simulink model "Lab2_3_sol"  (R2023b)
settings: Solver=VariableStepDiscrete  StartTime=0.0  StopTime=256*256*2  RelTol=1e-3  EnableMultiTasking=on
PreLoadFcn:
  | ImSize = 256;
undefined symbols (not defined in the file): gray, xc7k325tfbg676
libraries: hdlBasic x31, dspsigattribs x5, visionsources x1, vmcUtilities x1
settings Model: Creator=arvinds  LastModifiedBy=robg
settings SolverCC: AlgebraicLoopSolver=TrustRegion
settings DataIOCC: LimitDataPoints=on  SaveFormat=Array  SignalLoggingSaveFormat=ModelDataLogs  ReturnWorkspaceOutputs=off
settings OptimizationCC: ExpressionDepthLimit=2147483647  LifeSpan=inf
settings DebuggingCC: UnderspecifiedInitializationDetection=Classic  MergeDetectMultiDrivingBlocksExec=none  SolverPrmCheckMsg=warning  FcnCallInpInsideContextMsg=warning  UnconnectedInputMsg=warning  UnconnectedOutputMsg=warning  UnconnectedLineMsg=warning  AllowSymbolicDim=off  StateNameClashWarn=warning  SFUnexpectedBacktrackingDiag=warning  SFNoUnconditionalDefaultTransitionDiag=warning  SFExecutionAtInitializationDiag=none  ArithmeticOperatorsInVariantConditions=warning
settings HardwareCC: ProdBitPerPointer=32  ProdBitPerSizeT=32  ProdBitPerPtrDiffT=32  ProdLargestAtomicFloat=None  ProdIntDivRoundTo=Undefined  ProdEndianess=Unspecified  ProdWordSize=32  ProdHWDeviceType=32-bit Generic
settings ModelReferenceCC: EnableRefExpFcnMdlSchedulingChecks=on  PropagateSignalLabelsOutOfModel=off
settings SFSimCC: SimUseLocalCustomCode=off  CustomCodeUndefinedFunction=UseInterfaceOnly
settings RTWCC: RTWUseLocalCustomCode=off  DLArmComputeVersion=19.05
settings CodeAppCC: StateflowObjectComments=on
settings GRTTargetCC: TargetLangStandard=C89/C90 (ANSI)  CombineOutputUpdateFcns=off  GRTInterface=on
settings ConfigComp: CovMetricSettings=dw  CovSaveCumulativeToWorkspaceVar=on  CovSaveSingleToWorkspaceVar=on  CovExternalEMLEnable=off  CovSFcnEnable=off

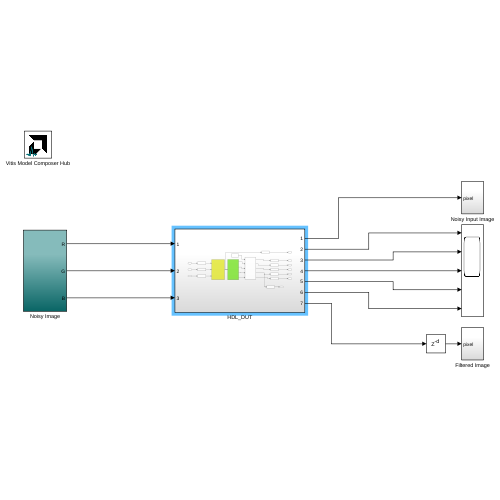
[thumbnail: Simulink's stored preview of the top-level diagram]
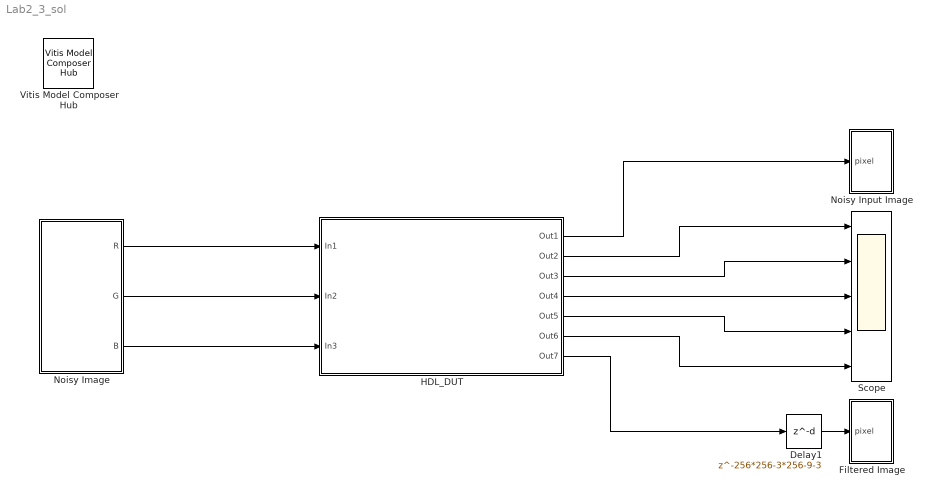
== system Lab2_3_sol ==
  Delay1 : Delay  DelayLength=256*256-3*256-9-3  SampleTime=1
  Filtered Image : Subsystem
  HDL_DUT : Subsystem
  Noisy Image : Subsystem
  Noisy Input Image : Subsystem
  Scope : Scope  NumInputPorts=5
  Vitis Model Composer Hub : vmcUtilities/Vitis Model Composer Hub  Tag=genX  CodeGeneration=off  SubsystemName=Lab2_3_sol  CompilationType=HDLCompilation  ExportTypeV2=IP Catalog  StartColumn=1  NumberOfColumns=1  TargetDirectory=./netlist  exportDesign=off  analyzeDesign=off  validateDesignOnHw=off  ExportType=System Generator  IpVendor=xilinx.com  IpLibrary=hls  IpVersion=1.0  IpHWLanguage=Verilog  AieCompilerOptions={}  AieSimulatorOptions={}  CreateTestbench=off  TestbenchStackSize=10  RunRtlSim=off  RunCSim=off  RunAieSim=off  AieSimTimeout=50000  RunAieSimProfiling=off  LaunchVitisAnalyzer=off  PlotOutput=off  RunX86Sim=off  X86SimTimeout=10  GenHwImage=off  GenLibadfXo=on  GenHwValidationCode=off  PlatformType=Not Specified  HwSystemType=Baremetal  HwValidationTarget=hw  ProjDevice=xc7k325tfbg676-3  ProjDevicePart=xc7k325tfbg676-3  SamplePeriod=-1  ClockFrequency=200  DataPathParallelism=1  xilinxfamily=kintex7  part=xc7k325t  speed=-3  package=fbg676  directory=./netlist/ip/Lab2_3_sol/src  testbench=off  incr_netlist=off  synthesis_tool=Vivado  clock_wrapper=Clock Enables  dbl_ovrd=According to Block Masks  dcm_input_clock_period=10  sysclk_period=5  simulink_period=1  eval_field=0  LogFileName=''  NThreads=4
  wires:
  Delay1/1 -> Filtered Image/1(pixel)
  Noisy Image/1(R) -> HDL_DUT/1(In1)
  Noisy Image/2(G) -> HDL_DUT/2(In2)
  Noisy Image/3(B) -> HDL_DUT/3(In3)
  HDL_DUT/1(Out1) -> Noisy Input Image/1(pixel)
  HDL_DUT/2(Out2) -> Scope/1
  HDL_DUT/3(Out3) -> Scope/2
  HDL_DUT/4(Out4) -> Scope/3
  HDL_DUT/5(Out5) -> Scope/4
  HDL_DUT/6(Out6) -> Scope/5
  HDL_DUT/7(Out7) -> Delay1/1

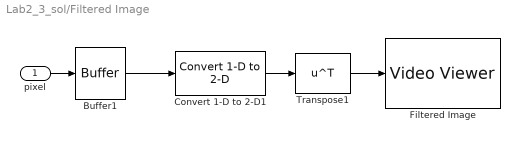
== system Lab2_3_sol/Filtered Image ==
  pixel : Inport
  Buffer1 : Buffer  N=ImSize*ImSize
  Convert 1-D to 2-D1 : dspsigattribs/Convert 1-D to 2-D  M=ImSize  N=ImSize  frameBasedOut=off
  Filtered Image : VideoViewer  colormapValue=gray(256)  FigPos=[721 702.8 408 300]
  Transpose1 : Math  Operator=transpose  SignedPower=on
  wires:
  Buffer1/1 -> Convert 1-D to 2-D1/1
  Convert 1-D to 2-D1/1 -> Transpose1/1
  pixel/1 -> Buffer1/1
  Transpose1/1 -> Filtered Image/1

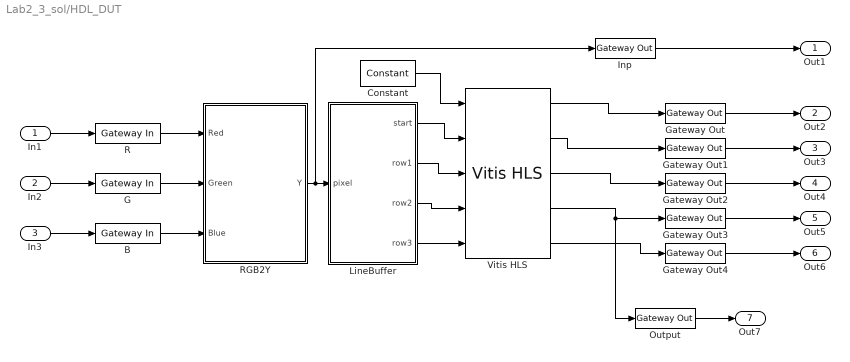
== system Lab2_3_sol/HDL_DUT ==
  In1 : Inport
  In2 : Inport  Port=2
  In3 : Inport  Port=3
  B : hdlBasic/Gateway In  gui_display_data_type=Fixed-point  arith_type=Unsigned  n_bits=8  bin_pt=0  preci_type=Single  exp_width=8  frac_width=24  rows=1  columns=1  quantization="Round  (unbiased: +/- Inf)"  overflow=Saturate  period=1  UseAsADC=off  ADCChannel='1'  interface=None  automatic_assignment=on  address_offset=hex2dec('00')  intf_name=''  intf_description=''  default_value=0  timing_constraint=None  locs_specified=off  LOCs={}  io_standard={}  inherit_from_input=off  hdl_port=on  XmcBlockStatus=1  maskContainerNames=group4  block_type=gatewayin  block_config=sysgen:gateway_in_config  block_width_w=590  block_height_w=620  block_width=640  block_height=850
  Constant : hdlBasic/Constant  const=0  gui_display_data_type=Boolean  arith_type=Boolean  n_bits=16  bin_pt=14  preci_type=Single  exp_width=8  frac_width=24  explicit_period=off  period=1  XmcBlockStatus=1  maskContainerNames=tabcontainer1  block_type=constant  block_config=sysgen:Constant_config
  G : hdlBasic/Gateway In  gui_display_data_type=Fixed-point  arith_type=Unsigned  n_bits=8  bin_pt=0  preci_type=Single  exp_width=8  frac_width=24  rows=1  columns=1  quantization="Round  (unbiased: +/- Inf)"  overflow=Saturate  period=1  UseAsADC=off  ADCChannel='1'  interface=None  automatic_assignment=on  address_offset=hex2dec('00')  intf_name=''  intf_description=''  default_value=0  timing_constraint=None  locs_specified=off  LOCs={}  io_standard={}  inherit_from_input=off  hdl_port=on  XmcBlockStatus=1  maskContainerNames=group4  block_type=gatewayin  block_config=sysgen:gateway_in_config  block_width_w=590  block_height_w=620  block_width=640  block_height=850
  Gateway Out{,1..4} (5 alike) : hdlBasic/Gateway Out  inherit_from_input=off  hdl_port=on  rows=1  columns=1  UseAsDAC=off  DACChannel='1'  interface=None  automatic_assignment=on  address_offset=hex2dec('00')  intf_name=''  intf_description=''  timing_constraint=None  locs_specified=off  LOCs={}  io_standard={}  XmcBlockStatus=1  maskContainerNames=group4  block_type=gatewayout  block_config=sysgen:gateway_out_config  block_width_w=590  block_height_w=620  block_width=620  block_height=750
  Inp : hdlBasic/Gateway Out  inherit_from_input=on  hdl_port=off  rows=1  columns=1  UseAsDAC=off  DACChannel='1'  interface=None  automatic_assignment=on  address_offset=hex2dec('00')  intf_name=''  intf_description=''  timing_constraint=None  locs_specified=off  LOCs={}  io_standard={}  XmcBlockStatus=1  maskContainerNames=group4  block_type=gatewayout  block_config=sysgen:gateway_out_config  block_width_w=590  block_height_w=620  block_width=620  block_height=750
  LineBuffer : Subsystem
  Output : hdlBasic/Gateway Out  inherit_from_input=on  hdl_port=on  rows=1  columns=1  UseAsDAC=off  DACChannel='1'  interface=None  automatic_assignment=on  address_offset=hex2dec('00')  intf_name=''  intf_description=''  timing_constraint=None  locs_specified=off  LOCs={}  io_standard={}  XmcBlockStatus=1  maskContainerNames=group4  block_type=gatewayout  block_config=sysgen:gateway_out_config  block_width_w=590  block_height_w=620  block_width=620  block_height=750
  R : hdlBasic/Gateway In  gui_display_data_type=Fixed-point  arith_type=Unsigned  n_bits=8  bin_pt=0  preci_type=Single  exp_width=8  frac_width=24  rows=1  columns=1  quantization="Round  (unbiased: +/- Inf)"  overflow=Saturate  period=1  UseAsADC=off  ADCChannel='1'  interface=None  automatic_assignment=on  address_offset=hex2dec('00')  intf_name=''  intf_description=''  default_value=0  timing_constraint=None  locs_specified=off  LOCs={}  io_standard={}  inherit_from_input=off  hdl_port=on  XmcBlockStatus=1  maskContainerNames=group4  block_type=gatewayin  block_config=sysgen:gateway_in_config  block_width_w=590  block_height_w=620  block_width=640  block_height=850
  RGB2Y : Subsystem
  Vitis HLS : hdlBasic/Vitis HLS  anytable='../hls_project/solution1'  fast_sim=off  display_datatype=off  rate_propagation_method=Simulink system period  model_file_path=''  latency=1  block_type=vitis_hls
      settings: infoedit=This block allows including C,C++ and SystemC source files in System Generator for DSP designs.
  Out1 : Outport
  Out2 : Outport  Port=2
  Out3 : Outport  Port=3
  Out4 : Outport  Port=4
  Out5 : Outport  Port=5
  Out6 : Outport  Port=6
  Out7 : Outport  Port=7
  wires:
  LineBuffer/3(row2) -> Vitis HLS/4
  Gateway Out/1 -> Out2/1
  Vitis HLS/2 -> Gateway Out1/1
  B/1 -> RGB2Y/3(Blue)
  Gateway Out1/1 -> Out3/1
  Constant/1 -> Vitis HLS/1
  In1/1 -> R/1
  Output/1 -> Out7/1
  R/1 -> RGB2Y/1(Red)
  Gateway Out4/1 -> Out6/1
  Vitis HLS/5 -> Gateway Out4/1
  Inp/1 -> Out1/1
  Gateway Out3/1 -> Out5/1
  RGB2Y/1(Y) -> LineBuffer/1(pixel), Inp/1
  LineBuffer/1(start) -> Vitis HLS/2
  Gateway Out2/1 -> Out4/1
  LineBuffer/4(row3) -> Vitis HLS/5
  G/1 -> RGB2Y/2(Green)
  Vitis HLS/1 -> Gateway Out/1
  In3/1 -> B/1
  LineBuffer/2(row1) -> Vitis HLS/3
  Vitis HLS/3 -> Gateway Out2/1
  In2/1 -> G/1
  Vitis HLS/4 -> Output/1, Gateway Out3/1

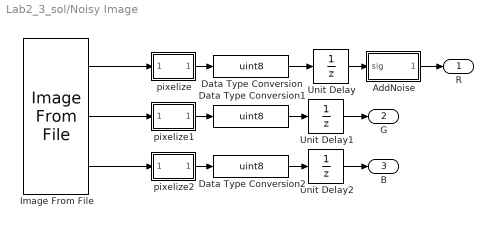
== system Lab2_3_sol/Noisy Image ==
  AddNoise : Subsystem
  Data Type Conversion : DataTypeConversion  OutDataTypeStr=uint8  SaturateOnIntegerOverflow=off  RndMeth=Floor
  Data Type Conversion1 : DataTypeConversion  OutDataTypeStr=uint8  SaturateOnIntegerOverflow=off  RndMeth=Floor
  Data Type Conversion2 : DataTypeConversion  OutDataTypeStr=uint8  SaturateOnIntegerOverflow=off  RndMeth=Floor
  Image From File : visionsources/Image From File  Tag=vipblks_nd  FileName=./xilinx_logo.jpg  Ts=ImSize*ImSize  imagePorts=Separate color signals  OutPortLabels=R|G|B  ImageDataType=uint8  sdImageDataType=uint(8)  Signed=on  WordLength=16  FractionLengthMode=User-defined  FractionLength=15
  Unit Delay : UnitDelay  SampleTime=-1  HasFrameUpgradeWarning=on
  Unit Delay1 : UnitDelay  SampleTime=-1  HasFrameUpgradeWarning=on
  Unit Delay2 : UnitDelay  SampleTime=-1  HasFrameUpgradeWarning=on
  pixelize : Subsystem
  pixelize1 : Subsystem
  pixelize2 : Subsystem
  R : Outport  VectorParamsAs1DForOutWhenUnconnected=off
  G : Outport  Port=2  VectorParamsAs1DForOutWhenUnconnected=off
  B : Outport  Port=3  VectorParamsAs1DForOutWhenUnconnected=off
  wires:
  Image From File/1 -> pixelize/1(In1)
  Data Type Conversion/1 -> Unit Delay/1
  pixelize/1(Out1) -> Data Type Conversion/1
  Data Type Conversion1/1 -> Unit Delay1/1
  pixelize1/1(Out1) -> Data Type Conversion1/1
  Image From File/2 -> pixelize1/1(In1)
  Data Type Conversion2/1 -> Unit Delay2/1
  pixelize2/1(Out1) -> Data Type Conversion2/1
  Image From File/3 -> pixelize2/1(In1)
  Unit Delay/1 -> AddNoise/1(sig)
  AddNoise/1(noise_sig) -> R/1
  Unit Delay1/1 -> G/1
  Unit Delay2/1 -> B/1

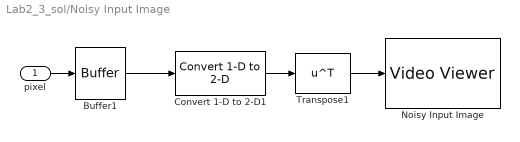
== system Lab2_3_sol/Noisy Input Image ==
  pixel : Inport
  Buffer1 : Buffer  N=ImSize*ImSize
  Convert 1-D to 2-D1 : dspsigattribs/Convert 1-D to 2-D  M=ImSize  N=ImSize  frameBasedOut=off
  Noisy Input Image : VideoViewer  colormapValue=gray(256)  FigPos=[286 708 420 293]
  Transpose1 : Math  Operator=transpose  SignedPower=on
  wires:
  Buffer1/1 -> Convert 1-D to 2-D1/1
  Convert 1-D to 2-D1/1 -> Transpose1/1
  pixel/1 -> Buffer1/1
  Transpose1/1 -> Noisy Input Image/1

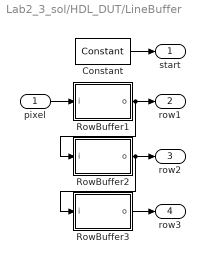
== system Lab2_3_sol/HDL_DUT/LineBuffer ==
  pixel : Inport
  Constant : hdlBasic/Constant  const=1  gui_display_data_type=Boolean  arith_type=Boolean  n_bits=16  bin_pt=14  preci_type=Single  exp_width=8  frac_width=24  explicit_period=off  period=1  XmcBlockStatus=1  maskContainerNames=tabcontainer1  block_type=constant  block_config=sysgen:Constant_config
  RowBuffer1 : Subsystem  mask(Virtex2 Line Buffer){buf_depth=ImSize, cst=1}
      mask prompts: buf_depth "Buffer Depth"; cst "Sample Period"
      mask help: The Xilinx Virtex2 Line Buffer reference block delayes a sequential stream of pixels by the specified buffer depth. It is optimized for the Virtex2 family since it uses the Read Before Write option on the underlying Single Port RAM block.
      mask init:
      | str = sprintf('-%d',buf_depth);
      | [bg,fg] = xlcmap('XBlock',0);
      | iPos = get_param(gcb,'Position');
      | iWidth=iPos(3)-iPos(1); iHeight=iPos(4)-iPos(2);
      | iCx=iWidth/2;
      | iCy=iHeight/2;
      | [logoX, logoY] = xlogo(iPos);
      mask Help: eval('');xlDoc('-book','sysgen','-topic','Virtex2_Line_Buffer');
      mask Display:
      | patch([0 iWidth iWidth 0],[0 0 iHeight iHeight] , bg);
      | patch(logoX,logoY , fg);
      | text(iCx-6,iCy,'z');
      | text(iCx,iCy+4,str);
      | plot([0 0 iWidth iWidth 0], [0 iHeight iHeight 0 0]);
  RowBuffer2 : Subsystem  mask(Virtex2 Line Buffer){buf_depth=ImSize, cst=1}
      mask prompts: buf_depth "Buffer Depth"; cst "Sample Period"
      mask help: The Xilinx Virtex2 Line Buffer reference block delayes a sequential stream of pixels by the specified buffer depth. It is optimized for the Virtex2 family since it uses the Read Before Write option on the underlying Single Port RAM block.
      mask init: same as Lab2_3_sol/HDL_DUT/LineBuffer/RowBuffer1
      mask Help: eval('');xlDoc('-book','sysgen','-topic','Virtex2_Line_Buffer');
      mask Display:
      | patch([0 iWidth iWidth 0],[0 0 iHeight iHeight] , bg);
      | patch(logoX,logoY , fg);
      | text(iCx-6,iCy,'z');
      | text(iCx,iCy+4,str);
      | plot([0 0 iWidth iWidth 0], [0 iHeight iHeight 0 0]);
  RowBuffer3 : Subsystem  mask(Virtex2 Line Buffer){buf_depth=ImSize, cst=1}
      mask prompts: buf_depth "Buffer Depth"; cst "Sample Period"
      mask help: The Xilinx Virtex2 Line Buffer reference block delayes a sequential stream of pixels by the specified buffer depth. It is optimized for the Virtex2 family since it uses the Read Before Write option on the underlying Single Port RAM block.
      mask init: same as Lab2_3_sol/HDL_DUT/LineBuffer/RowBuffer1
      mask Help: eval('');xlDoc('-book','sysgen','-topic','Virtex2_Line_Buffer');
      mask Display:
      | patch([0 iWidth iWidth 0],[0 0 iHeight iHeight] , bg);
      | patch(logoX,logoY , fg);
      | text(iCx-6,iCy,'z');
      | text(iCx,iCy+4,str);
      | plot([0 0 iWidth iWidth 0], [0 iHeight iHeight 0 0]);
  start : Outport  VectorParamsAs1DForOutWhenUnconnected=off
  row1 : Outport  Port=2  VectorParamsAs1DForOutWhenUnconnected=off
  row2 : Outport  Port=3  VectorParamsAs1DForOutWhenUnconnected=off
  row3 : Outport  Port=4  VectorParamsAs1DForOutWhenUnconnected=off
  wires:
  RowBuffer1/1(o) -> RowBuffer2/1(i), row1/1
  RowBuffer2/1(o) -> RowBuffer3/1(i), row2/1
  pixel/1 -> RowBuffer1/1(i)
  RowBuffer3/1(o) -> row3/1
  Constant/1 -> start/1

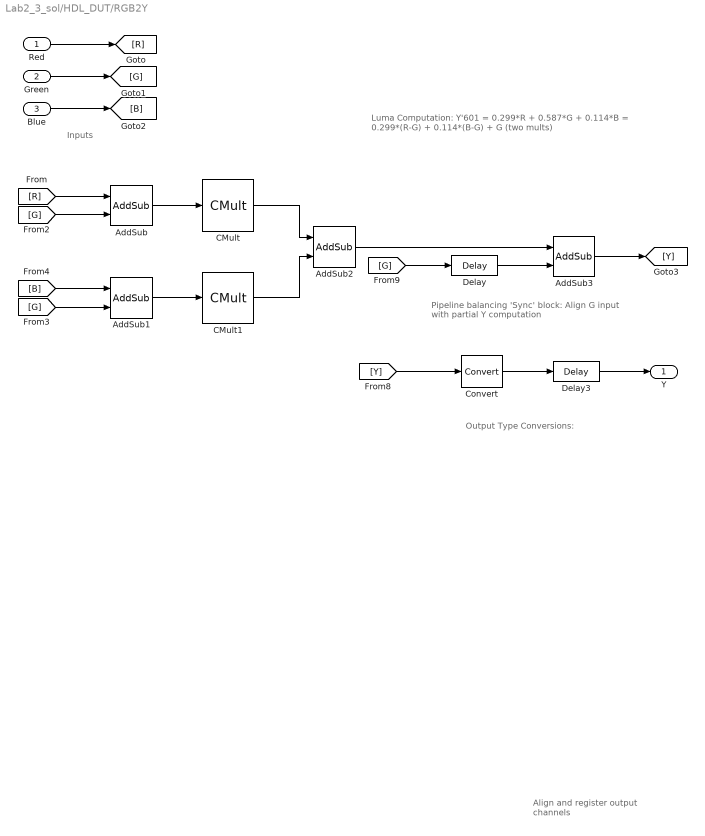
== system Lab2_3_sol/HDL_DUT/RGB2Y ==
  note: Luma Computation:
      |
      |  Y'601 = 0.299*R + 0.587*G + 0.114*B
      |           = 0.299*(R-G) + 0.114*(B-G) + G   (two mults)
  note: Inputs
  note: Pipeline balancing 'Sync' block:
      | Align G input with partial Y computation
  note: Align and register
      | output channels
  note: Output Type Conversions:
  Red : Inport
  Green : Inport  Port=2
  Blue : Inport  Port=3
  AddSub : hdlBasic/AddSub  mode=Subtraction  use_carryin=off  use_carryout=off  en=off  latency=1  precision=Full  arith_type=Unsigned  n_bits=8  bin_pt=2  quantization=Truncate  overflow=Wrap  use_behavioral_HDL=off  hw_selection=Fabric  pipelined=off  use_rpm=off  XmcBlockStatus=1  maskContainerNames=tabcontainer1  block_type=addsub  block_config=sysgen:Addsub_config
  AddSub1 : hdlBasic/AddSub  mode=Subtraction  use_carryin=off  use_carryout=off  en=off  latency=1  precision=Full  arith_type=Unsigned  n_bits=8  bin_pt=2  quantization=Truncate  overflow=Wrap  use_behavioral_HDL=off  hw_selection=Fabric  pipelined=off  use_rpm=off  XmcBlockStatus=1  maskContainerNames=tabcontainer1  block_type=addsub  block_config=sysgen:Addsub_config
  AddSub2 : hdlBasic/AddSub  mode=Addition  use_carryin=off  use_carryout=off  en=off  latency=1  precision=Full  arith_type=Unsigned  n_bits=8  bin_pt=2  quantization=Truncate  overflow=Wrap  use_behavioral_HDL=off  hw_selection=Fabric  pipelined=off  use_rpm=off  XmcBlockStatus=1  maskContainerNames=tabcontainer1  block_type=addsub  block_config=sysgen:Addsub_config
  AddSub3 : hdlBasic/AddSub  mode=Addition  use_carryin=off  use_carryout=off  en=off  latency=1  precision=User Defined  arith_type="Signed  (2's comp)"  n_bits=10  bin_pt=0  quantization="Round  (unbiased: +/- Inf)"  overflow=Saturate  use_behavioral_HDL=off  hw_selection=Fabric  pipelined=off  use_rpm=off  XmcBlockStatus=1  maskContainerNames=tabcontainer1  block_type=addsub  block_config=sysgen:Addsub_config
  CMult : hdlBasic/CMult  const=0.299  gui_display_data_type=Fixed-point  const_n_bits=12  const_bin_pt=12  float_type=Single  exp_bits=8  fraction_bits=24  en=off  latency=3  precision=Full  arith_type="Signed  (2's comp)"  n_bits=8  bin_pt=2  quantization="Round  (unbiased: +/- Inf)"  overflow=Wrap  use_behavioral_HDL=off  mem_type=Distributed RAM  pipeline=off  use_rpm=off  placement_style=Triangular Packing  XmcBlockStatus=1  maskContainerNames=tabcontainer1  block_type=cmult  block_config=sysgen:CMult_config
      settings: infoedit=[]
  CMult1 : hdlBasic/CMult  const=0.114  gui_display_data_type=Fixed-point  const_n_bits=12  const_bin_pt=12  float_type=Single  exp_bits=8  fraction_bits=24  en=off  latency=3  precision=Full  arith_type="Signed  (2's comp)"  n_bits=8  bin_pt=2  quantization="Round  (unbiased: +/- Inf)"  overflow=Wrap  use_behavioral_HDL=off  mem_type=Distributed RAM  pipeline=off  use_rpm=off  placement_style=Triangular Packing  XmcBlockStatus=1  maskContainerNames=tabcontainer1  block_type=cmult  block_config=sysgen:CMult_config
      settings: infoedit=[]
  Convert : hdlBasic/Convert  gui_display_data_type=Fixed-point  arith_type=Unsigned  n_bits=8  bin_pt=0  float_type=Single  exp_bits=8  fraction_bits=24  quantization="Round  (unbiased: +/- Inf)"  overflow=Saturate  en=off  latency=0  pipeline=off  XmcBlockStatus=1  maskContainerNames=group2  block_type=convert  block_config=sysgen:Convert_config  block_width=595  block_height=885
  Delay : hdlBasic/Delay  rst=off  en=off  latency=5  reg_retiming=off  XmcBlockStatus=1  maskContainerNames=group1  block_type=delay  block_config=sysgen:Delay_config
  Delay3 : hdlBasic/Delay  rst=off  en=off  latency=5  reg_retiming=off  XmcBlockStatus=1  maskContainerNames=group1  block_type=delay  block_config=sysgen:Delay_config
  Y : Outport  VectorParamsAs1DForOutWhenUnconnected=off
  wires:
  [G] -> AddSub/2
  [G] -> Delay/1
  Delay/1 -> AddSub3/2
  AddSub3/1 -> [Y]
  [B] -> AddSub1/1
  [G] -> AddSub1/2
  [R] -> AddSub/1
  Blue/1 -> [B]
  Green/1 -> [G]
  Red/1 -> [R]
  [Y] -> Convert/1
  CMult/1 -> AddSub2/1
  CMult1/1 -> AddSub2/2
  AddSub/1 -> CMult/1
  AddSub1/1 -> CMult1/1
  AddSub2/1 -> AddSub3/1
  Delay3/1 -> Y/1
  Convert/1 -> Delay3/1

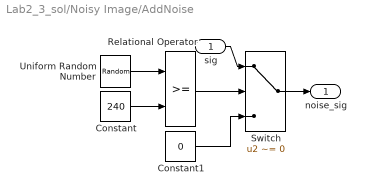
== system Lab2_3_sol/Noisy Image/AddNoise ==
  sig : Inport
  Constant : Constant  Value=240
  Constant1 : Constant  Value=0
  Relational Operator : RelationalOperator  OutDataTypeStr=boolean  SampleTime=1  InputSameDT=off
  Switch : Switch  Criteria=u2 ~= 0  SampleTime=1  SaturateOnIntegerOverflow=off  InputSameDT=off
  Uniform Random Number : UniformRandomNumber  Minimum=0  Maximum=255  SampleTime=1
  noise_sig : Outport  VectorParamsAs1DForOutWhenUnconnected=off
  wires:
  Uniform Random Number/1 -> Relational Operator/1
  Relational Operator/1 -> Switch/2
  Constant/1 -> Relational Operator/2
  Constant1/1 -> Switch/3
  sig/1 -> Switch/1
  Switch/1 -> noise_sig/1

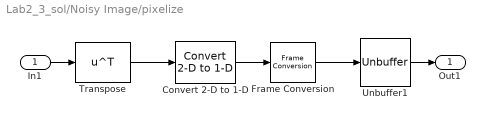
== system Lab2_3_sol/Noisy Image/pixelize ==
  In1 : Inport
  Convert 2-D to 1-D : dspsigattribs/Convert 2-D to 1-D
  Frame Conversion : FrameConversion
  Transpose : Math  Operator=transpose  SignedPower=on
  Unbuffer1 : Unbuffer
  Out1 : Outport  VectorParamsAs1DForOutWhenUnconnected=off
  wires:
  Convert 2-D to 1-D/1 -> Frame Conversion/1
  Frame Conversion/1 -> Unbuffer1/1
  Transpose/1 -> Convert 2-D to 1-D/1
  In1/1 -> Transpose/1
  Unbuffer1/1 -> Out1/1

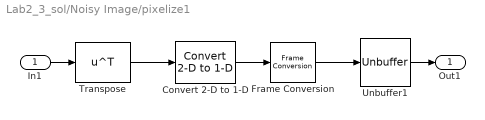
== system Lab2_3_sol/Noisy Image/pixelize1 ==
  In1 : Inport
  Convert 2-D to 1-D : dspsigattribs/Convert 2-D to 1-D
  Frame Conversion : FrameConversion
  Transpose : Math  Operator=transpose  SignedPower=on
  Unbuffer1 : Unbuffer
  Out1 : Outport  VectorParamsAs1DForOutWhenUnconnected=off
  wires:
  Unbuffer1/1 -> Out1/1
  In1/1 -> Transpose/1
  Transpose/1 -> Convert 2-D to 1-D/1
  Frame Conversion/1 -> Unbuffer1/1
  Convert 2-D to 1-D/1 -> Frame Conversion/1

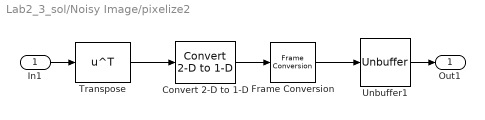
== system Lab2_3_sol/Noisy Image/pixelize2 ==
  In1 : Inport
  Convert 2-D to 1-D : dspsigattribs/Convert 2-D to 1-D
  Frame Conversion : FrameConversion
  Transpose : Math  Operator=transpose  SignedPower=on
  Unbuffer1 : Unbuffer
  Out1 : Outport  VectorParamsAs1DForOutWhenUnconnected=off
  wires:
  Convert 2-D to 1-D/1 -> Frame Conversion/1
  Frame Conversion/1 -> Unbuffer1/1
  Transpose/1 -> Convert 2-D to 1-D/1
  In1/1 -> Transpose/1
  Unbuffer1/1 -> Out1/1

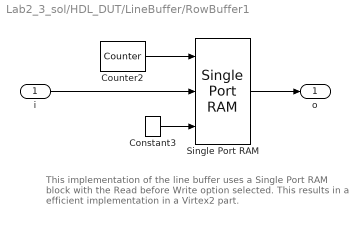
== system Lab2_3_sol/HDL_DUT/LineBuffer/RowBuffer1 ==
  note: This implementation of the line buffer uses a
      |  Single Port RAM block with the Read before Write
      | option selected.  This results in a efficient
      | implementation in a Virtex2 part.
  i : Inport
  Constant3 : hdlBasic/Constant  const=1  gui_display_data_type=Boolean  arith_type=Boolean  n_bits=1  bin_pt=0  preci_type=Single  exp_width=8  frac_width=24  explicit_period=on  period=cst  XmcBlockStatus=1  maskContainerNames=tabcontainer1  block_type=constant  block_config=sysgen:Constant_config
  Counter2 : hdlBasic/Counter  cnt_type=Count limited  cnt_to=buf_depth -2  operation=Up  start_count=0  cnt_by_val=1  arith_type=Unsigned  n_bits=ceil(log2(buf_depth-1))  bin_pt=0  load_pin=off  rst=off  en=off  explicit_period=Explicit  period=cst  use_behavioral_HDL=off  implementation=Fabric  XmcBlockStatus=1  maskContainerNames=group1  block_type=counter  block_config=sysgen:Counter_config  block_width=531  block_height=1023
  Single Port RAM : hdlBasic/Single Port RAM  depth=buf_depth-1  initVector=0  distributed_mem=Block RAM  write_mode=Read Before Write  rst=off  init_reg=0  en=off  optimize_latency=off  latency=1  optimize=Area  dbl_ovrd=off  simulation_type=fast_sim  XmcBlockStatus=1  maskContainerNames=tabcontainer1  block_type=spram  block_config=sysgen:SPRAM_config
      settings: xl_area=[0 0 1 0 0 0 0]
  o : Outport  VectorParamsAs1DForOutWhenUnconnected=off
  wires:
  Constant3/1 -> Single Port RAM/3
  Single Port RAM/1 -> o/1
  i/1 -> Single Port RAM/2
  Counter2/1 -> Single Port RAM/1

== system Lab2_3_sol/HDL_DUT/LineBuffer/RowBuffer2 ==
  note: This implementation of the line buffer uses a
      |  Single Port RAM block with the Read before Write
      | option selected.  This results in a efficient
      | implementation in a Virtex2 part.
  i : Inport
  Constant3 : hdlBasic/Constant  const=1  gui_display_data_type=Boolean  arith_type=Boolean  n_bits=1  bin_pt=0  preci_type=Single  exp_width=8  frac_width=24  explicit_period=on  period=cst  XmcBlockStatus=1  maskContainerNames=tabcontainer1  block_type=constant  block_config=sysgen:Constant_config
  Counter2 : hdlBasic/Counter  cnt_type=Count limited  cnt_to=buf_depth -2  operation=Up  start_count=0  cnt_by_val=1  arith_type=Unsigned  n_bits=ceil(log2(buf_depth-1))  bin_pt=0  load_pin=off  rst=off  en=off  explicit_period=Explicit  period=cst  use_behavioral_HDL=off  implementation=Fabric  XmcBlockStatus=1  maskContainerNames=group1  block_type=counter  block_config=sysgen:Counter_config  block_width=531  block_height=1023
  Single Port RAM : hdlBasic/Single Port RAM  depth=buf_depth-1  initVector=0  distributed_mem=Block RAM  write_mode=Read Before Write  rst=off  init_reg=0  en=off  optimize_latency=off  latency=1  optimize=Area  dbl_ovrd=off  simulation_type=fast_sim  XmcBlockStatus=1  maskContainerNames=tabcontainer1  block_type=spram  block_config=sysgen:SPRAM_config
      settings: xl_area=[0 0 1 0 0 0 0]
  o : Outport  VectorParamsAs1DForOutWhenUnconnected=off
  wires:
  Counter2/1 -> Single Port RAM/1
  i/1 -> Single Port RAM/2
  Single Port RAM/1 -> o/1
  Constant3/1 -> Single Port RAM/3

== system Lab2_3_sol/HDL_DUT/LineBuffer/RowBuffer3 ==
  note: This implementation of the line buffer uses a
      |  Single Port RAM block with the Read before Write
      | option selected.  This results in a efficient
      | implementation in a Virtex2 part.
  i : Inport
  Constant3 : hdlBasic/Constant  const=1  gui_display_data_type=Boolean  arith_type=Boolean  n_bits=1  bin_pt=0  preci_type=Single  exp_width=8  frac_width=24  explicit_period=on  period=cst  XmcBlockStatus=1  maskContainerNames=tabcontainer1  block_type=constant  block_config=sysgen:Constant_config
  Counter2 : hdlBasic/Counter  cnt_type=Count limited  cnt_to=buf_depth -2  operation=Up  start_count=0  cnt_by_val=1  arith_type=Unsigned  n_bits=ceil(log2(buf_depth-1))  bin_pt=0  load_pin=off  rst=off  en=off  explicit_period=Explicit  period=cst  use_behavioral_HDL=off  implementation=Fabric  XmcBlockStatus=1  maskContainerNames=group1  block_type=counter  block_config=sysgen:Counter_config  block_width=531  block_height=1023
  Single Port RAM : hdlBasic/Single Port RAM  depth=buf_depth-1  initVector=0  distributed_mem=Block RAM  write_mode=Read Before Write  rst=off  init_reg=0  en=off  optimize_latency=off  latency=1  optimize=Area  dbl_ovrd=off  simulation_type=fast_sim  XmcBlockStatus=1  maskContainerNames=tabcontainer1  block_type=spram  block_config=sysgen:SPRAM_config
      settings: xl_area=[0 0 1 0 0 0 0]
  o : Outport  VectorParamsAs1DForOutWhenUnconnected=off
  wires:
  Constant3/1 -> Single Port RAM/3
  Single Port RAM/1 -> o/1
  i/1 -> Single Port RAM/2
  Counter2/1 -> Single Port RAM/1
